simulink model "Integration_relay"  (Simulink 8.1)
settings: Solver=ode4  StartTime=0.0  StopTime=inf  FixedStep=Ts  MaxStep=1e-3  RelTol=1e-3
model workspace (MAT data in the model file):
  op_snapshot1 : opcond.OperatingPoint (value not decoded)
PostLoadFcn:
  | Ts=100e-6; HILLTOP_init;
InitFcn:
  | Ts=100e-6; HILLTOP_init;
undefined symbols (not defined in the file): F1, Left, type, V
libraries: rtlab x6, artemis x5, cables_lib x3, breaker_lib x2, Load_lib x2, powerlib x2, transformer_lib x2, relay_modbus_lib x2, ssn_lib x1
settings Model: ARTEMISmethode_block_infos=$$__separator__$$Integration_relay/ARTEMIS Guide$$__separator__$$  Creator=RE25624  LastModifiedBy=re25624  BufferReuse=off
settings SolverCC: ZeroCrossAlgorithm=Adaptive
settings DataIOCC: ExternalInput=getinputstruct(op_snapshot1)  InitialState=getstatestruct(op_snapshot1)  LimitDataPoints=off  MaxDataPoints=90060  SignalLoggingSaveFormat=Dataset  SaveOutput=off  SignalLogging=off  DSMLogging=off  SaveTime=off  OutputSaveName=result
settings OptimizationCC: BlockReduction=off  OptimizeBlockIOStorage=off  BufferReuse=off  ExpressionFolding=off  LocalBlockOutputs=off
settings DebuggingCC: MaxConsecutiveZCsMsg=warning  IgnoredZcDiagnostic=none  SolverPrmCheckMsg=none  MultiTaskRateTransMsg=warning  FcnCallInpInsideContextMsg=EnableAllAsWarning  FrameProcessingCompatibilityMsg=error  ModelReferenceExtraNoncontSigs=warning  StrictBusMsg=None
settings ModelReferenceCC: UpdateModelReferenceTargets=IfOutOfDate
settings SFSimCC: SFSimEcho=off
settings GRTTargetCC: CodeReplacementLibrary=C89/C90 (ANSI)

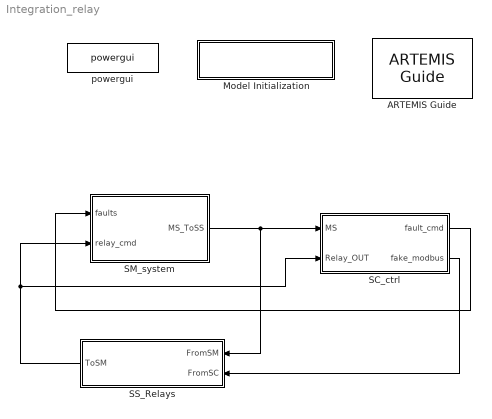
== system Integration_relay ==
  ARTEMIS Guide : artemis/ARTEMIS/ARTEMIS Guide  Tag=FTSSmethode_opal_4hx0r99  Description=5.0_z1  lock=on  Ts=Ts  opt=art5  dyna=off  nb_perm=4  RT_fullcomp=off  ssn=on  ssn_itvc=off  ssn_ivic=off  ssn_ext=off  ssn_solver=Art5 with Backward Euler nodal interface  ssn_impulse=off  ssn_quasimpulse=off  ssn_impulse_loop=2  paraExtinctionThy=off  Thy_Impulse=on  dtc=Off  dtc_opt=normal  ao=on  simtype=off  ct_mac=off  lin_mov=off  lsp=[0.001 2]  spike_skip=Disabled  dtc_extra=1  dtc_sws=normal  dtc_pied=0.5  SPSRulesBlock=SPSRules  tre=on  ctmm=off  LF=off  dpl_type=ARTEMiS DPL  rlc_type=off  custom_type=off  para=on  ssn_ImpulseLoopBlockedStateUpdate=2  ssn_mov_iter_number=5  ssn_switch_iter_number=5
  Model Initialization : Subsystem  AncestorBlock=artemis/Tools /Misc/Model Initialization  mask(Model Functions){InitFcnX=Ts=100e-6; HILLTOP_init;, prel=off, posl=on, inif=on, strf=off}
      mask prompts: InitFcnX "Initialisation"; prel "Preload Function"; posl "PostLoad Function"; inif "InitFcn"; strf "StartFcn"
      mask init:
      | currentBlock = gcb;
      | root = bdroot(currentBlock);
      | 
      | if ~strcmp(get_param(root,'BlockDiagramType'),'library')
      |     if prel==1
      |         set_param(root, 'PreLoadFcn', InitFcnX);
      |     else
      |         set_param(root, 'PreLoadFcn', '');
      |     end
      |     if inif==1
      |         set_param(root, 'InitFcn', InitFcnX);
      |     else
      |         set_param(root, 'InitFcn', '');
      |     end
      |     if strf==1
      |         set_param(root, 'StartFcn', InitFcnX);
      |     else
      |         set_param(root, 'StartFcn', '');
      |     end
      |     if posl==1
      |         set_param(root, 'PostLoadFcn', InitFcnX);
      |     else
      |         set_param(root, 'PostLoadFcn', '');
      |     end
      | end
      | 
      | pos = get_param(currentBlock, 'Position');
      | width = pos(3) - pos(1); height = pos(4) - pos(2);
      | txt = [ upper(root) '\n' '- InitFcn. . . . . '  get_param(root, 'InitFcn') ];
      settings: CopyFcn=set_param(gcb,'LinkStatus','inactive')
      mask Display: text(5, height*0.5, txt, 'horizontalAlignment', 'left', 'verticalAlignment', 'middle') ;
  SC_ctrl : Subsystem
  SM_system : Subsystem
  SS_Relays : Subsystem
  powergui : powerlib/powergui  Priority=2  SimulationMode=Discrete  SolverType=Tustin  SampleTime=Ts  frequency=60  SPID=off  DisableSnubberDevices=off  DisableRonSwitches=off  DisableVfSwitches=off  SwTol=0  Interpol=off  DisplayEquations=off  frequencyindice=0  Pbase=100e6  ErrMax=1e-4  Iterations=50  UnitsV=kV  UnitsW=MW  FunctionMessages=off  echomessages=off  HookPort=off  EnableUseOfTLC=off  x0status=blocks  RestoreLinks=warning  ResistiveCurrentMeasurement=off  Frange=logspace(0,3,50)  Ylog=off  Xlog=off  ShowGrid=off  save=off  variable=ZData  structure=0  ZoomFFT=on  StartTime=0.0  cycles=2  DisplayStyle=off  fundamental=60  FreqAxis=off  MaxFrequency=1000  frequencyindicesteady=1  RmsSteady=1  display=off  Ts=0  methode=off
  wires:
  SM_system/1(MS_ToSS) -> SS_Relays/1(FromSM), SC_ctrl/1(MS)
  SC_ctrl/1(fault_cmd) -> SM_system/1(faults)
  SS_Relays/1(ToSM) -> SC_ctrl/2(Relay_OUT), SM_system/2(relay_cmd)
  SC_ctrl/2(fake_modbus) -> SS_Relays/2(FromSC)

== system Integration_relay/Model Initialization ==

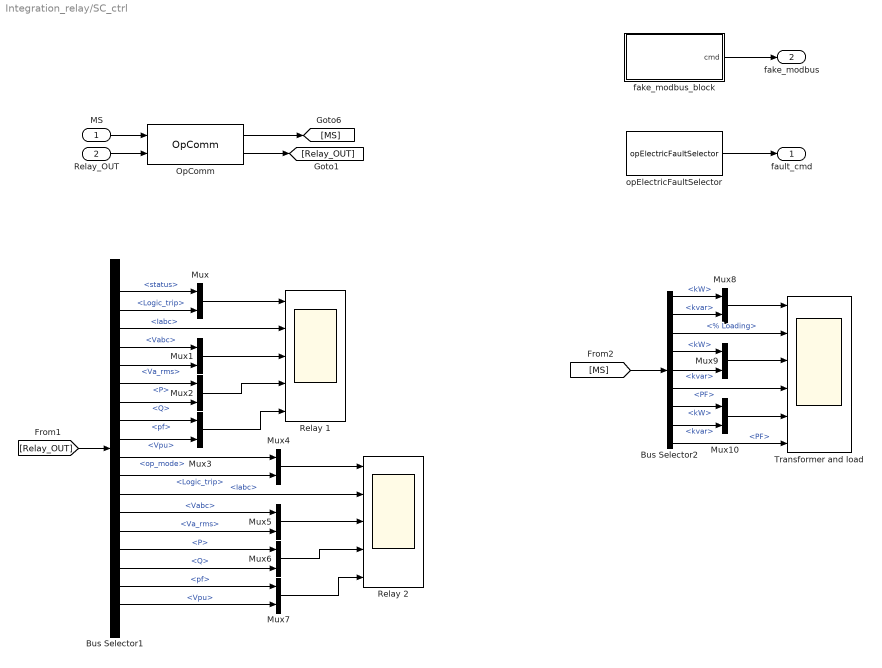
== system Integration_relay/SC_ctrl ==
  MS : Inport
  Relay_OUT : Inport  Port=2
  Bus Selector1 : BusSelector  OutputSignals=relay_1.m.status,relay_1.Logic_trip,relay_1.m.Iabc,relay_1.m.Vabc,relay_1.m.Va_rms,relay_1.m.P,relay_1.m.Q,relay_1.m.pf,relay_1.m.Vpu,relay_2.op_mode,relay_2.Logic_trip,relay_2.m.Iabc,relay_2.m.Vabc,relay_2.m.Va_rms,relay_2.m.P,relay_2.m.Q,relay_2.m.pf,relay_2.m.Vpu
  Bus Selector2 : BusSelector  OutputSignals=xfr_activeLoad.kW,xfr_activeLoad.kvar,xfr_activeLoad.% Loading,load_1.kW,load_1.kvar,load_1.PF,load_2.kW,load_2.kvar,load_2.PF
  Mux{,1..10} (11 alike) : Mux  Inputs=2
  OpComm : rtlab/OpComm  nbport=2  groupe_acq=1  subsys_rate=0  st=0  Synchronization=on  Interpolation=on  Threshold=1.0  Missed_Data=off  Sim_Time=off  Samples=off  dynSigOut=off  from_console=0  warning_done=off  writeOpCommFile=off  Offset=off
  Relay 1 : Scope  NumInputPorts=5
      settings: ShowLegends=on  TimeRange=0.4  YMin=9.494623655913976~-150~-15000~-500000~0  YMax=17.49462365591398~200~15000~2000000~1.4  SaveName=ScopeData2
  Relay 2 : Scope  NumInputPorts=5
      settings: ShowLegends=on  TimeRange=1  YMin=0~-3000~-4000~-200000~0  YMax=1~2000~4000~1000000~2.5  SaveName=ScopeData4
  Transformer and load : Scope  NumInputPorts=6
      settings: ShowLegends=on  TimeRange=30  YMin=0~0~0~0~0~0  YMax=1000~1000~1000~1250~1000~1.3  SaveName=ScopeData3
  fake_modbus_block : Subsystem  mask(Fake Modbus Command){a=0, b=0, c=0, d=0, e=0, f=0}
      mask prompts: a "Relay#1: Reset"; b "Relay#1: Mode"; c "Relay#1: Group Settings"; d "Relay#2: Reset"; e "Relay#2: Mode"; f "Relay#2: Group Settings"
  opElectricFaultSelector : artemis/Tools /POW faults/opElectricFaultSelector  phase_a=on  phase_b=on  phase_c=on  gnd_fault=on  Tacq=1  Tst=[0.1 0 10]  enable_POW=off  angle_POW=[15 0 10]  Tdr="[0.5 0  10]"  fault_location_menu=No fault  T_init=2
  fault_cmd : Outport
  fake_modbus : Outport  Port=2
  wires:
  OpComm/1 -> [MS]
  MS/1 -> OpComm/1
  opElectricFaultSelector/1 -> fault_cmd/1
  [Relay_OUT] -> Bus Selector1/1
  OpComm/2 -> [Relay_OUT]
  Relay_OUT/1 -> OpComm/2
  [MS] -> Bus Selector2/1
  Bus Selector1/3 -> Relay 1/2  "<Iabc>"
  Bus Selector1/1 -> Mux/1  "<status>"
  Bus Selector1/2 -> Mux/2  "<Logic_trip>"
  Bus Selector1/4 -> Mux1/1  "<Vabc>"
  Bus Selector1/5 -> Mux1/2  "<Va_rms>"
  Bus Selector1/6 -> Mux2/1  "<P>"
  Bus Selector1/7 -> Mux2/2  "<Q>"
  Bus Selector1/8 -> Mux3/1  "<pf>"
  Bus Selector1/9 -> Mux3/2  "<Vpu>"
  Mux/1 -> Relay 1/1
  Mux1/1 -> Relay 1/3
  Mux2/1 -> Relay 1/4
  Mux3/1 -> Relay 1/5
  Bus Selector1/12 -> Relay 2/2  "<Iabc>"
  Bus Selector1/10 -> Mux4/1  "<op_mode>"
  Bus Selector1/11 -> Mux4/2  "<Logic_trip>"
  Bus Selector1/13 -> Mux5/1  "<Vabc>"
  Bus Selector1/14 -> Mux5/2  "<Va_rms>"
  Bus Selector1/15 -> Mux6/1  "<P>"
  Bus Selector1/16 -> Mux6/2  "<Q>"
  Bus Selector1/17 -> Mux7/1  "<pf>"
  Bus Selector1/18 -> Mux7/2  "<Vpu>"
  Mux4/1 -> Relay 2/1
  Mux5/1 -> Relay 2/3
  Mux6/1 -> Relay 2/4
  Mux7/1 -> Relay 2/5
  Bus Selector2/1 -> Mux8/1  "<kW>"
  Bus Selector2/2 -> Mux8/2  "<kvar>"
  Bus Selector2/3 -> Transformer and load/2  "<% Loading>"
  Bus Selector2/4 -> Mux9/1  "<kW>"
  Bus Selector2/5 -> Mux9/2  "<kvar>"
  Bus Selector2/6 -> Transformer and load/4  "<PF>"
  Bus Selector2/7 -> Mux10/1  "<kW>"
  Bus Selector2/8 -> Mux10/2  "<kvar>"
  Bus Selector2/9 -> Transformer and load/6  "<PF>"
  Mux8/1 -> Transformer and load/1
  Mux9/1 -> Transformer and load/3
  Mux10/1 -> Transformer and load/5
  fake_modbus_block/1(cmd) -> fake_modbus/1

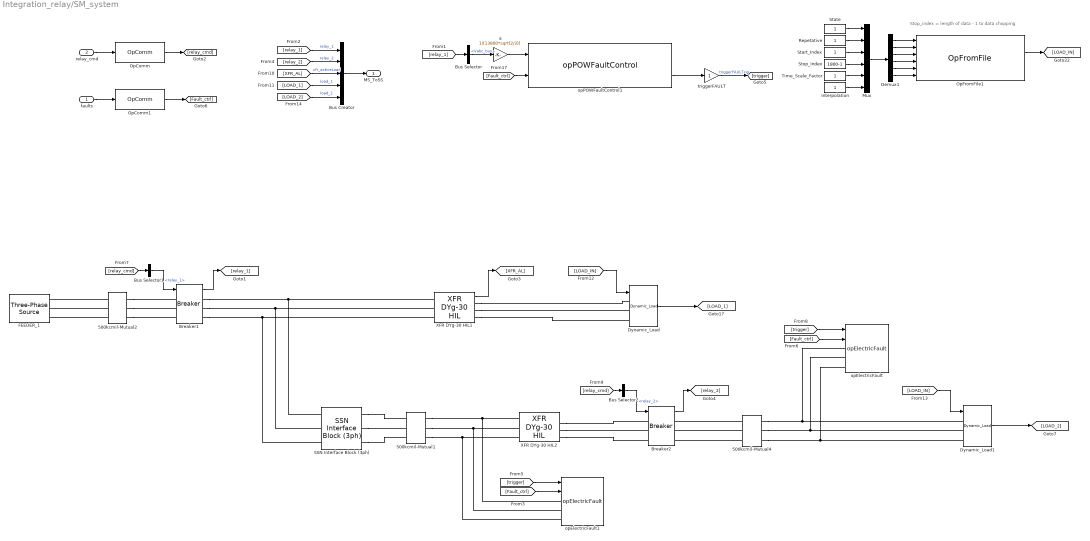
== system Integration_relay/SM_system ==
  note: Stop_index = length of data - 1 to data chopping
  faults : Inport
  relay_cmd : Inport  Port=2
  500kcmil-Mutual1 : cables_lib/500kcmil-Mutual  length=5000  par_sets=1  ratio=3
  500kcmil-Mutual2 : cables_lib/500kcmil-Mutual  length=5000  par_sets=1  ratio=3
  500kcmil-Mutual4 : cables_lib/500kcmil-Mutual  length=1100  par_sets=1  ratio=3
  Breaker1 : breaker_lib/Breaker  Ts=Ts
  Breaker2 : breaker_lib/Breaker  Ts=Ts
  Bus Creator : BusCreator  Inputs=5
  Bus Selector : BusSelector  OutputSignals=Vabc_bus
  Bus Selector1 : BusSelector  OutputSignals=relay_1
  Bus Selector2 : BusSelector  OutputSignals=relay_2
  Demux1 : Demux  Outputs=6
  Dynamic_Load : Load_lib/Dynamic_Load  V=460  P_Scale=1  Q_Scale=1  kVA_min=10  PF_avg=0.90
  Dynamic_Load1 : Load_lib/Dynamic_Load  V=460  P_Scale=1  Q_Scale=1  kVA_min=10  PF_avg=0.90
  FEEDER_1 : powerlib/Electrical Sources/Three-Phase Source  Voltage=13800  PhaseAngle=0  Frequency=60  InternalConnection=Yg  SpecifyImpedance=on  Resistance=0.8929  Inductance=16.58e-3  ShortCircuitLevel=375e6  BaseVoltage=13800  XRratio=7.9  BusType=swing  Pref=0  Qref=0  Qmin=-inf  Qmax=inf
  "Interpolation " : Constant
  Mux : Mux  Inputs=6
  OpComm : rtlab/OpComm  nbport=1  groupe_acq=1  subsys_rate=0  st=0  Synchronization=on  Interpolation=on  Threshold=1.0  Missed_Data=off  Sim_Time=off  Samples=off  dynSigOut=off  from_console=0  warning_done=off  writeOpCommFile=off  Offset=off
  OpComm1 : rtlab/OpComm  nbport=1  groupe_acq=1  subsys_rate=0  st=0  Synchronization=on  Interpolation=on  Threshold=1.0  Missed_Data=off  Sim_Time=off  Samples=off  dynSigOut=off  from_console=1  warning_done=off  writeOpCommFile=off  Offset=off
  OpFromFile1 : rtlab/DataLogging/OpFromFile  filename_mode=Static (same filename all the time)  reload_mode=Next time model is paused (Real-Time)  init_file_id=0  filename=one_min_data.mat  rtpath='./'  nrtpath='.\'  sample_time=0
  "Repetative " : Constant
  SSN Interface Block (3ph) : ssn_lib/SSN Interface Block (3ph)  nb_phase=3  nb_port=2  p1_type=V-type(Left)  p2_type=V-type (Right)  p3_type=V-type(Left)  p4_type=V-type(Left)  p5_type=V-type(Left)  p6_type=V-type(Left)  p7_type=V-type(Left)  p8_type=V-type(Left)  p9_type=V-type(Left)  p10_type=V-type(Left)  p11_type=V-type(Left)  p12_type=V-type(Left)  p13_type=V-type(Left)  p14_type=V-type(Left)  p15_type=V-type(Left)  p16_type=V-type(Left)  I_port_shunt_resistance=1e9
  "Start_Index " : Constant
  "State " : Constant
  "Stop_Index " : Constant  Value=1800-1
  "Time_Scale_Factor " : Constant
  XFR DYg-30 HIL1 : transformer_lib/XFR DYg-30 HIL  Rating=2500  Vp=13800  Vs=480  Z=5.18  XR=2.5
  XFR DYg-30 HIL2 : transformer_lib/XFR DYg-30 HIL  Rating=2500  Vp=13800  Vs=460  Z=5.18  XR=2.5
  a : Gain  Gain=1/(13800*sqrt(2/3))
  opElectricFault : artemis/Tools /POW faults/opElectricFault  FaultLocation=location 2  FaultResistance=0.0001  GroundResistance=0.0001  InitialStates=[0 0 0]  SnubberResistance=1e6  SnubberCapacitance=inf
  opElectricFault1 : artemis/Tools /POW faults/opElectricFault  FaultLocation=location 1  FaultResistance=0.0001  GroundResistance=0.0001  InitialStates=[0 0 0]  SnubberResistance=1e6  SnubberCapacitance=inf
  opPOWFaultControl1 : artemis/Tools /POW faults/opPOWFaultControl  Ts=Ts  usePLL=off  Fgrid=60  PLL_k=[180 3200 1]  vol_sel=1: rising zero-corssing  SyncPhase_menu=A  T_acq=0.8
  triggerFAULT : Gain
  MS_ToSS : Outport
  wires:
  Breaker1/1 -> [relay_1]
  [Fault_ctrl] -> opPOWFaultControl1/2
  opPOWFaultControl1/2 -> triggerFAULT/1
  triggerFAULT/1 -> [trigger]  "triggerFAULTsig"
  [Fault_ctrl] -> opElectricFault/2
  [trigger] -> opElectricFault/1
  [relay_1] -> Bus Selector/1
  Bus Selector/1 -> a/1  "<Vabc_bus>"
  a/1 -> opPOWFaultControl1/1
  Breaker2/1 -> [relay_2]
  [Fault_ctrl] -> opElectricFault1/2
  [trigger] -> opElectricFault1/1
  [relay_1] -> Bus Creator/1  "relay_1"
  [relay_2] -> Bus Creator/2  "relay_2"
  Bus Creator/1 -> MS_ToSS/1
  [relay_cmd] -> Bus Selector1/1
  Bus Selector1/1 -> Breaker1/1  "<relay_1>"
  [relay_cmd] -> Bus Selector2/1
  Bus Selector2/1 -> Breaker2/1  "<relay_2>"
  OpComm/1 -> [relay_cmd]
  OpComm1/1 -> [Fault_ctrl]
  faults/1 -> OpComm1/1
  relay_cmd/1 -> OpComm/1
  Dynamic_Load/1 -> [LOAD_1]
  "Stop_Index "/1 -> Mux/4
  Demux1/2 -> OpFromFile1/2
  Demux1/5 -> OpFromFile1/5
  OpFromFile1/2 -> [LOAD_IN]
  "Interpolation "/1 -> Mux/6
  Mux/1 -> Demux1/1
  Demux1/4 -> OpFromFile1/4
  Demux1/1 -> OpFromFile1/1
  Demux1/6 -> OpFromFile1/6
  Demux1/3 -> OpFromFile1/3
  "Start_Index "/1 -> Mux/3
  "Time_Scale_Factor "/1 -> Mux/5
  "Repetative "/1 -> Mux/2
  "State "/1 -> Mux/1
  XFR DYg-30 HIL1/1 -> [XFR_AL]
  [LOAD_1] -> Bus Creator/4  "load_1"
  [XFR_AL] -> Bus Creator/3  "xfr_activeLoad"
  [LOAD_IN] -> Dynamic_Load/1
  Dynamic_Load1/1 -> [LOAD_2]
  [LOAD_IN] -> Dynamic_Load1/1
  [LOAD_2] -> Bus Creator/5  "load_2"
  connections:
  500kcmil-Mutual2/LConn2 -- FEEDER_1/RConn2
  500kcmil-Mutual2/LConn1 -- FEEDER_1/RConn1
  500kcmil-Mutual2/LConn3 -- FEEDER_1/RConn3
  500kcmil-Mutual4/RConn2 -- Dynamic_Load1/LConn2 -- opElectricFault/LConn2
  500kcmil-Mutual4/RConn1 -- Dynamic_Load1/LConn1 -- opElectricFault/LConn1
  500kcmil-Mutual4/RConn3 -- Dynamic_Load1/LConn3 -- opElectricFault/LConn3
  opElectricFault1/LConn1 -- 500kcmil-Mutual1/RConn1 -- XFR DYg-30 HIL2/LConn1
  opElectricFault1/LConn2 -- 500kcmil-Mutual1/RConn2 -- XFR DYg-30 HIL2/LConn2
  opElectricFault1/LConn3 -- 500kcmil-Mutual1/RConn3 -- XFR DYg-30 HIL2/LConn3
  500kcmil-Mutual2/RConn1 -- Breaker1/LConn1
  500kcmil-Mutual2/RConn2 -- Breaker1/LConn2
  500kcmil-Mutual2/RConn3 -- Breaker1/LConn3
  500kcmil-Mutual4/LConn1 -- Breaker2/RConn1
  500kcmil-Mutual4/LConn2 -- Breaker2/RConn2
  500kcmil-Mutual4/LConn3 -- Breaker2/RConn3
  XFR DYg-30 HIL2/RConn2 -- Breaker2/LConn2
  XFR DYg-30 HIL2/RConn1 -- Breaker2/LConn1
  XFR DYg-30 HIL2/RConn3 -- Breaker2/LConn3
  Breaker1/RConn1 -- SSN Interface Block (3ph)/LConn1 -- XFR DYg-30 HIL1/LConn1
  Breaker1/RConn2 -- SSN Interface Block (3ph)/LConn2 -- XFR DYg-30 HIL1/LConn2
  Breaker1/RConn3 -- SSN Interface Block (3ph)/LConn3 -- XFR DYg-30 HIL1/LConn3
  XFR DYg-30 HIL1/RConn2 -- Dynamic_Load/LConn2
  XFR DYg-30 HIL1/RConn1 -- Dynamic_Load/LConn1
  XFR DYg-30 HIL1/RConn3 -- Dynamic_Load/LConn3
  SSN Interface Block (3ph)/RConn2 -- 500kcmil-Mutual1/LConn2
  SSN Interface Block (3ph)/RConn1 -- 500kcmil-Mutual1/LConn1
  SSN Interface Block (3ph)/RConn3 -- 500kcmil-Mutual1/LConn3

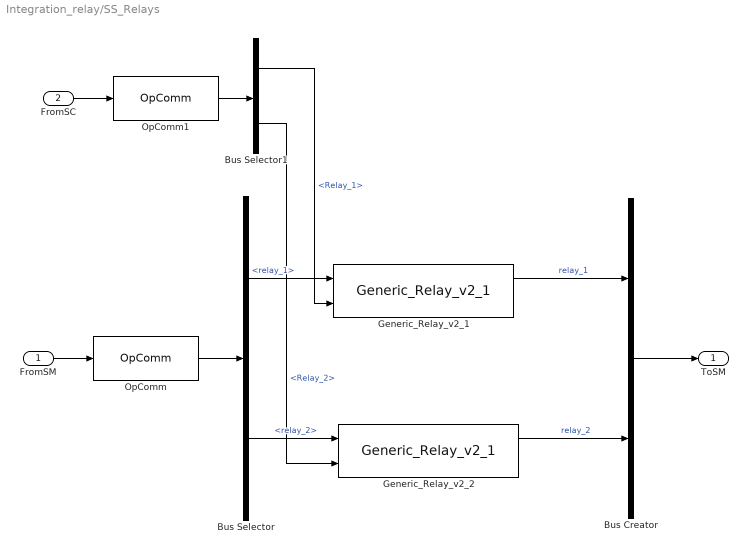
== system Integration_relay/SS_Relays ==
  FromSM : Inport
  FromSC : Inport  Port=2
  Bus Creator : BusCreator  Inputs=2
  Bus Selector : BusSelector  OutputSignals=relay_1,relay_2
  Bus Selector1 : BusSelector  OutputSignals=Relay_1,Relay_2
  Generic_Relay_v2_1 : relay_modbus_lib/Generic_Relay_v2_1  bkrCtrl_enable=0  bkrCtrl_status=1  Ts=Ts  relay_settings=[F1(1,:)]
  Generic_Relay_v2_2 : relay_modbus_lib/Generic_Relay_v2_1  bkrCtrl_enable=0  bkrCtrl_status=1  Ts=Ts  relay_settings=[F1(2,:)]
  OpComm : rtlab/OpComm  nbport=1  groupe_acq=1  subsys_rate=0  st=0  Synchronization=on  Interpolation=on  Threshold=1.0  Missed_Data=off  Sim_Time=off  Samples=off  dynSigOut=off  from_console=0  warning_done=off  writeOpCommFile=off  Offset=off
  OpComm1 : rtlab/OpComm  nbport=1  groupe_acq=1  subsys_rate=0  st=0  Synchronization=on  Interpolation=on  Threshold=1.0  Missed_Data=off  Sim_Time=off  Samples=off  dynSigOut=off  from_console=1  warning_done=off  writeOpCommFile=off  Offset=off
  ToSM : Outport
  wires:
  OpComm/1 -> Bus Selector/1
  FromSM/1 -> OpComm/1
  Bus Selector/1 -> Generic_Relay_v2_1/1  "<relay_1>"
  Bus Selector/2 -> Generic_Relay_v2_2/1  "<relay_2>"
  Generic_Relay_v2_1/1 -> Bus Creator/1  "relay_1"
  Generic_Relay_v2_2/1 -> Bus Creator/2  "relay_2"
  Bus Creator/1 -> ToSM/1
  FromSC/1 -> OpComm1/1
  OpComm1/1 -> Bus Selector1/1
  Bus Selector1/2 -> Generic_Relay_v2_2/2  "<Relay_2>"
  Bus Selector1/1 -> Generic_Relay_v2_1/2  "<Relay_1>"

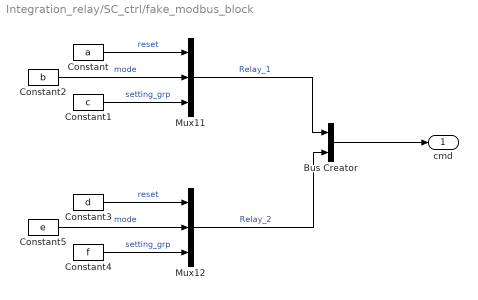
== system Integration_relay/SC_ctrl/fake_modbus_block ==
  Bus Creator : BusCreator  Inputs=2
  Constant : Constant  Value=a
  Constant1 : Constant  Value=c
  Constant2 : Constant  Value=b
  Constant3 : Constant  Value=d
  Constant4 : Constant  Value=f
  Constant5 : Constant  Value=e
  Mux11 : Mux  Inputs=3
  Mux12 : Mux  Inputs=3
  cmd : Outport
  wires:
  Bus Creator/1 -> cmd/1
  Mux11/1 -> Bus Creator/1  "Relay_1"
  Constant5/1 -> Mux12/2  "mode"
  Constant4/1 -> Mux12/3  "setting_grp"
  Constant3/1 -> Mux12/1  "reset"
  Mux12/1 -> Bus Creator/2  "Relay_2"
  Constant1/1 -> Mux11/3  "setting_grp"
  Constant2/1 -> Mux11/2  "mode"
  Constant/1 -> Mux11/1  "reset"
